simulink model "full_maneuver_platoon_new_strategy"  (R2019a)
settings: Solver=VariableStepAuto  StartTime=0.0  StopTime=70  FixedStep=0.1  MaxStep=0.05  RelTol=1e-3
libraries: simulink x97, dspsigops x7, powerlib_meascontrol x7, autolibshared x7
(part 2 of 7)

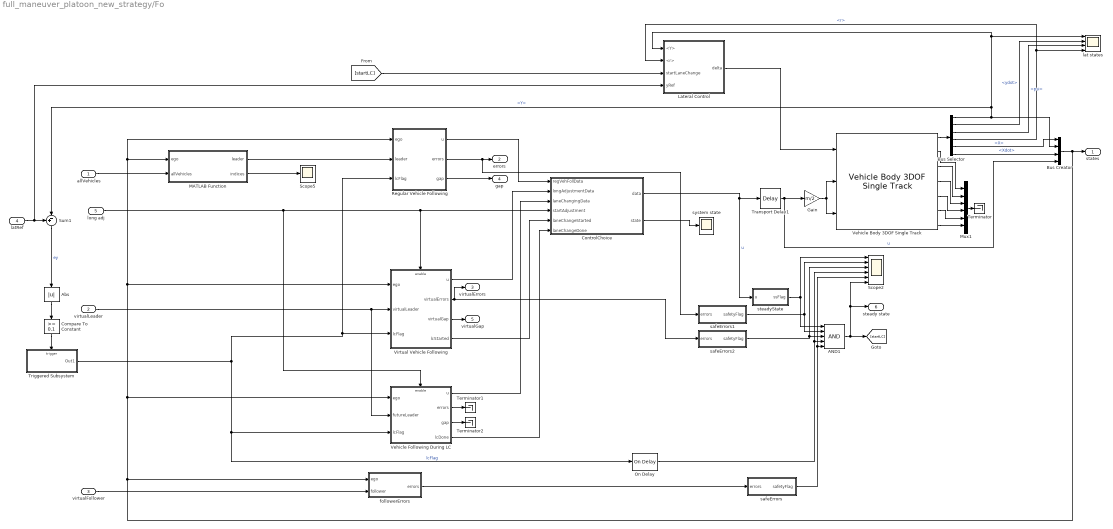
== system full_maneuver_platoon_new_strategy/Fo ==
  allVehicles : Inport
  virtualLeader : Inport  Port=2
  virtualFollower : Inport  Port=3
  latRef : Inport  Port=4
  long adj : Inport  Port=5
  AND1 : Logic  Inputs=5  IconShape=distinctive  AllPortsSameDT=off  OutDataTypeStr=boolean
  Abs : Abs
  Bus Creator : BusCreator  Inputs=4  OutDataTypeStr=Bus: vehStatesBus  NonVirtualBus=on
  Bus Selector : BusSelector  OutputSignals=InertFrm.Cg.Disp.Y,BdyFrm.Cg.Vel.ydot,InertFrm.Cg.Ang.psi,BdyFrm.Cg.AngVel.r,InertFrm.RearAxl.Disp.X,InertFrm.RearAxl.Vel.Xdot
  Compare To Constant : simulink/Logic and Bit Operations/Compare To Constant  relop=>=  const=0.1  OutDataTypeStr=boolean
  ControlChoice : Stateflow chart  BlockKeywords=__PRM__SERIALIZED__DATA__:Stateflow Chart,Stateflow Diagram  TreatAsAtomicUnit=on
  Gain : Gain  Gain=m/2
  Lateral Control : Subsystem
  MATLAB Function : MATLAB Function  TreatAsAtomicUnit=on
  Mux1 : Mux  Inputs=6
  On Delay : powerlib_meascontrol/Logic/On Delay  DelayType=On delay  delay=1  ic=0  Ts=0
      settings: SourceProductName=Simscape Electrical
  Regular Vehicle Following : Subsystem
  Scope2 : Scope  NumInputPorts=6
  Scope5 : Scope
  Sum1 : Sum  Inputs=+-|
  Terminator : Terminator
  Terminator1 : Terminator
  Terminator2 : Terminator
  Transport Delay1 : TransportDelay  DelayTime=0.01
  Triggered Subsystem : Subsystem  TreatAsAtomicUnit=on
  Vehicle Body 3DOF Single Track : autolibshared/Vehicle Body 3DOF Single Track  trackMode=Single (bicycle)  inputMode=External longitudinal forces  frontSteerMode=on  rearSteerMode=off  windMode=off  muMode=off  extFMode=off  extMMode=off  extXo=off  extpsio=off  extxdoto=off  extro=off  extYo=off  extTamb=off  extydoto=off  aMode=2  NF=2  NR=2  m=m  a=lf  b=lr  h=0.35  X_o=x0  xdot_o=vx0  CalphaMode=off  sigmaMode=on  d=0  w=[1.4,1.4]  Cy_f=12e3  Cy_r=11e3  sigma_f=.1  sigma_r=.1  alpha_f_brk=[-.1 .1]  Cy_f_data=[-9e3 9e3]  alpha_r_brk=[-.1 .1]  Cy_r_data=[-9e3 9e3]  Y_o=y0  ydot_o=0  Izz=4000  psi_o=0  r_o=0  Af=2  Cd=.3  Cl=.1  Cpm=.1  beta_w=[0:0.01:0.3]  Cs=[0:0.03:0.9]  Cym=[0:0.01:0.3]  Pabs=101325  Tair=273  g=9.81  mu=1  xdot_tol=.01  Fznom=5000  Fxtire_sat=7e4  Fytire_sat=7e4  longOff=0  latOff=0  vertOff=0  wrapAng=off
      settings: SourceProductName=Powertrain Blockset  SourceProductBaseCode=PW
  Vehicle Following During LC : Subsystem  TreatAsAtomicUnit=on
  Virtual Vehicle Following : Subsystem  TreatAsAtomicUnit=on
  followerErrors : Subsystem
  lat states : Scope  NumInputPorts=4
  safeErrors : Subsystem
  safeErrors1 : Subsystem
  safeErrors2 : Subsystem
  steadyState : Subsystem
  system state : Scope
  states : Outport
  errors : Outport  Port=2
  virtualErrors : Outport  Port=3
  gap : Outport  Port=4
  virtualGap : Outport  Port=5
  steady state : Outport  Port=6
  wires:
  Virtual Vehicle Following/2(virtualErrors) -> safeErrors2/1(errors), virtualErrors/1
  Sum1/1 -> Abs/1  "ey"
  Transport Delay1/1 -> Gain/1, Bus Creator/4  "u"
  virtualLeader/1 -> Vehicle Following During LC/2(futureLeader), Virtual Vehicle Following/2(virtualLeader)
  On Delay/1 -> Scope2/4, AND1/4
  long adj/1 -> Vehicle Following During LC/Enable, Virtual Vehicle Following/Enable, ControlChoice/4(startAdjustment)
  AND1/1 -> Scope2/6, steady state/1, [startLC]
  Bus Creator/1 -> states/1, Regular Vehicle Following/1(ego), MATLAB Function/1(ego), Virtual Vehicle Following/1(ego), Vehicle Following During LC/1(ego), followerErrors/1(ego)
  ControlChoice/1(data) -> Transport Delay1/1, steadyState/1(u)  "u"
  latRef/1 -> Lateral Control/4(yRef), Sum1/1
  Bus Selector/4 -> Lateral Control/2(<r>), lat states/4  "<r>"
  Bus Selector/3 -> lat states/3  "<psi>"
  Bus Selector/2 -> lat states/2  "<ydot>"
  Bus Selector/1 -> Lateral Control/1(<Y>), lat states/1, Sum1/2, Bus Creator/2  "<Y>"
  Mux1/1 -> Terminator/1
  Vehicle Body 3DOF Single Track/7 -> Mux1/6
  Vehicle Body 3DOF Single Track/6 -> Mux1/5
  Vehicle Body 3DOF Single Track/5 -> Mux1/4
  Vehicle Body 3DOF Single Track/2 -> Mux1/1
  Vehicle Body 3DOF Single Track/3 -> Mux1/2
  Vehicle Body 3DOF Single Track/4 -> Mux1/3
  Vehicle Body 3DOF Single Track/1 -> Bus Selector/1
  Gain/1 -> Vehicle Body 3DOF Single Track/2, Vehicle Body 3DOF Single Track/3
  Bus Selector/5 -> Bus Creator/1  "<X>"
  Bus Selector/6 -> Bus Creator/3  "<Xdot>"
  Triggered Subsystem/1(Out1) -> On Delay/1, Vehicle Following During LC/3(lcFlag), Regular Vehicle Following/3(lcFlag), Virtual Vehicle Following/3(lcFlag)  "lcFlag"
  Abs/1 -> Compare To Constant/1
  Compare To Constant/1 -> Triggered Subsystem/Trigger
  allVehicles/1 -> MATLAB Function/2(allVehicles)
  MATLAB Function/1(leader) -> Regular Vehicle Following/2(leader)
  safeErrors/1(safetyFlag) -> Scope2/5, AND1/5
  followerErrors/1(errors) -> safeErrors/1(errors)
  safeErrors1/1(safetyFlag) -> AND1/2, Scope2/2
  safeErrors2/1(safetyFlag) -> AND1/3, Scope2/3
  steadyState/1(ssFlag) -> AND1/1, Scope2/1
  virtualFollower/1 -> followerErrors/2(follower)
  MATLAB Function/2(indices) -> Scope5/1
  Regular Vehicle Following/3(gap) -> gap/1
  Regular Vehicle Following/1(u) -> ControlChoice/1(regVehFollData)
  Virtual Vehicle Following/1(u) -> ControlChoice/2(longAdjustmentData)
  Regular Vehicle Following/2(errors) -> safeErrors1/1(errors), errors/1
  [startLC] -> Lateral Control/3(startLaneChange)
  Lateral Control/1(delta) -> Vehicle Body 3DOF Single Track/1
  Virtual Vehicle Following/4(lcStarted) -> ControlChoice/5(laneChangeStarted)
  ControlChoice/2(state) -> system state/1
  Vehicle Following During LC/1(u) -> ControlChoice/3(laneChangingData)
  Vehicle Following During LC/4(lcDone) -> ControlChoice/6(laneChangeDone)
  Vehicle Following During LC/2(errors) -> Terminator1/1
  Vehicle Following During LC/3(gap) -> Terminator2/1
  Virtual Vehicle Following/3(virtualGap) -> virtualGap/1

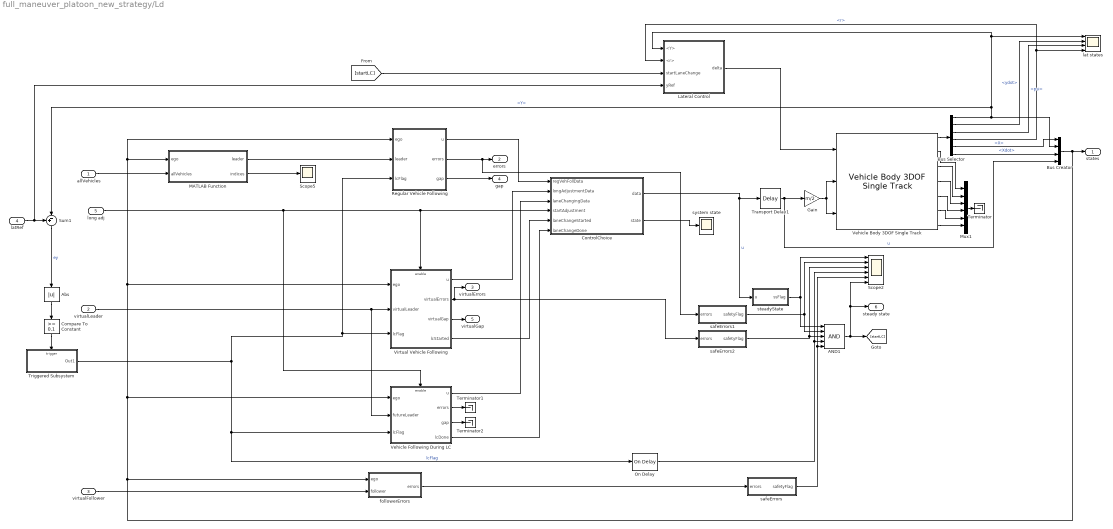
== system full_maneuver_platoon_new_strategy/Ld ==
  allVehicles : Inport
  virtualLeader : Inport  Port=2
  virtualFollower : Inport  Port=3
  latRef : Inport  Port=4
  long adj : Inport  Port=5
  AND1 : Logic  Inputs=5  IconShape=distinctive  AllPortsSameDT=off  OutDataTypeStr=boolean
  Abs : Abs
  Bus Creator : BusCreator  Inputs=4  OutDataTypeStr=Bus: vehStatesBus  NonVirtualBus=on
  Bus Selector : BusSelector  OutputSignals=InertFrm.Cg.Disp.Y,BdyFrm.Cg.Vel.ydot,InertFrm.Cg.Ang.psi,BdyFrm.Cg.AngVel.r,InertFrm.RearAxl.Disp.X,InertFrm.RearAxl.Vel.Xdot
  Compare To Constant : simulink/Logic and Bit Operations/Compare To Constant  relop=>=  const=0.1  OutDataTypeStr=boolean
  ControlChoice : Stateflow chart  BlockKeywords=__PRM__SERIALIZED__DATA__:Stateflow Chart,Stateflow Diagram  TreatAsAtomicUnit=on
  Gain : Gain  Gain=m/2
  Lateral Control : Subsystem
  MATLAB Function : MATLAB Function  TreatAsAtomicUnit=on
  Mux1 : Mux  Inputs=6
  On Delay : powerlib_meascontrol/Logic/On Delay  DelayType=On delay  delay=1  ic=0  Ts=0
      settings: SourceProductName=Simscape Electrical
  Regular Vehicle Following : Subsystem
  Scope2 : Scope  NumInputPorts=6
  Scope5 : Scope
  Sum1 : Sum  Inputs=+-|
  Terminator : Terminator
  Terminator1 : Terminator
  Terminator2 : Terminator
  Transport Delay1 : TransportDelay  DelayTime=0.01
  Triggered Subsystem : Subsystem  TreatAsAtomicUnit=on
  Vehicle Body 3DOF Single Track : autolibshared/Vehicle Body 3DOF Single Track  trackMode=Single (bicycle)  inputMode=External longitudinal forces  frontSteerMode=on  rearSteerMode=off  windMode=off  muMode=off  extFMode=off  extMMode=off  extXo=off  extpsio=off  extxdoto=off  extro=off  extYo=off  extTamb=off  extydoto=off  aMode=2  NF=2  NR=2  m=m  a=lf  b=lr  h=0.35  X_o=x0  xdot_o=vx0  CalphaMode=off  sigmaMode=on  d=0  w=[1.4,1.4]  Cy_f=12e3  Cy_r=11e3  sigma_f=.1  sigma_r=.1  alpha_f_brk=[-.1 .1]  Cy_f_data=[-9e3 9e3]  alpha_r_brk=[-.1 .1]  Cy_r_data=[-9e3 9e3]  Y_o=y0  ydot_o=0  Izz=4000  psi_o=0  r_o=0  Af=2  Cd=.3  Cl=.1  Cpm=.1  beta_w=[0:0.01:0.3]  Cs=[0:0.03:0.9]  Cym=[0:0.01:0.3]  Pabs=101325  Tair=273  g=9.81  mu=1  xdot_tol=.01  Fznom=5000  Fxtire_sat=7e4  Fytire_sat=7e4  longOff=0  latOff=0  vertOff=0  wrapAng=off
      settings: SourceProductName=Powertrain Blockset  SourceProductBaseCode=PW
  Vehicle Following During LC : Subsystem  TreatAsAtomicUnit=on
  Virtual Vehicle Following : Subsystem  TreatAsAtomicUnit=on
  followerErrors : Subsystem
  lat states : Scope  NumInputPorts=4
  safeErrors : Subsystem
  safeErrors1 : Subsystem
  safeErrors2 : Subsystem
  steadyState : Subsystem
  system state : Scope
  states : Outport
  errors : Outport  Port=2
  virtualErrors : Outport  Port=3
  gap : Outport  Port=4
  virtualGap : Outport  Port=5
  steady state : Outport  Port=6
  wires:
  Virtual Vehicle Following/2(virtualErrors) -> safeErrors2/1(errors), virtualErrors/1
  Sum1/1 -> Abs/1  "ey"
  Transport Delay1/1 -> Gain/1, Bus Creator/4  "u"
  virtualLeader/1 -> Vehicle Following During LC/2(futureLeader), Virtual Vehicle Following/2(virtualLeader)
  On Delay/1 -> Scope2/4, AND1/4
  long adj/1 -> Vehicle Following During LC/Enable, Virtual Vehicle Following/Enable, ControlChoice/4(startAdjustment)
  AND1/1 -> Scope2/6, steady state/1, [startLC]
  Bus Creator/1 -> states/1, Regular Vehicle Following/1(ego), MATLAB Function/1(ego), Virtual Vehicle Following/1(ego), Vehicle Following During LC/1(ego), followerErrors/1(ego)
  ControlChoice/1(data) -> Transport Delay1/1, steadyState/1(u)  "u"
  latRef/1 -> Lateral Control/4(yRef), Sum1/1
  Bus Selector/4 -> Lateral Control/2(<r>), lat states/4  "<r>"
  Bus Selector/3 -> lat states/3  "<psi>"
  Bus Selector/2 -> lat states/2  "<ydot>"
  Bus Selector/1 -> Lateral Control/1(<Y>), lat states/1, Sum1/2, Bus Creator/2  "<Y>"
  Mux1/1 -> Terminator/1
  Vehicle Body 3DOF Single Track/7 -> Mux1/6
  Vehicle Body 3DOF Single Track/6 -> Mux1/5
  Vehicle Body 3DOF Single Track/5 -> Mux1/4
  Vehicle Body 3DOF Single Track/2 -> Mux1/1
  Vehicle Body 3DOF Single Track/3 -> Mux1/2
  Vehicle Body 3DOF Single Track/4 -> Mux1/3
  Vehicle Body 3DOF Single Track/1 -> Bus Selector/1
  Gain/1 -> Vehicle Body 3DOF Single Track/2, Vehicle Body 3DOF Single Track/3
  Bus Selector/5 -> Bus Creator/1  "<X>"
  Bus Selector/6 -> Bus Creator/3  "<Xdot>"
  Triggered Subsystem/1(Out1) -> On Delay/1, Vehicle Following During LC/3(lcFlag), Regular Vehicle Following/3(lcFlag), Virtual Vehicle Following/3(lcFlag)  "lcFlag"
  Abs/1 -> Compare To Constant/1
  Compare To Constant/1 -> Triggered Subsystem/Trigger
  allVehicles/1 -> MATLAB Function/2(allVehicles)
  MATLAB Function/1(leader) -> Regular Vehicle Following/2(leader)
  safeErrors/1(safetyFlag) -> Scope2/5, AND1/5
  followerErrors/1(errors) -> safeErrors/1(errors)
  safeErrors1/1(safetyFlag) -> AND1/2, Scope2/2
  safeErrors2/1(safetyFlag) -> AND1/3, Scope2/3
  steadyState/1(ssFlag) -> AND1/1, Scope2/1
  virtualFollower/1 -> followerErrors/2(follower)
  MATLAB Function/2(indices) -> Scope5/1
  Regular Vehicle Following/3(gap) -> gap/1
  Regular Vehicle Following/1(u) -> ControlChoice/1(regVehFollData)
  Virtual Vehicle Following/1(u) -> ControlChoice/2(longAdjustmentData)
  Regular Vehicle Following/2(errors) -> safeErrors1/1(errors), errors/1
  [startLC] -> Lateral Control/3(startLaneChange)
  Lateral Control/1(delta) -> Vehicle Body 3DOF Single Track/1
  Virtual Vehicle Following/4(lcStarted) -> ControlChoice/5(laneChangeStarted)
  ControlChoice/2(state) -> system state/1
  Vehicle Following During LC/1(u) -> ControlChoice/3(laneChangingData)
  Vehicle Following During LC/4(lcDone) -> ControlChoice/6(laneChangeDone)
  Vehicle Following During LC/2(errors) -> Terminator1/1
  Vehicle Following During LC/3(gap) -> Terminator2/1
  Virtual Vehicle Following/3(virtualGap) -> virtualGap/1

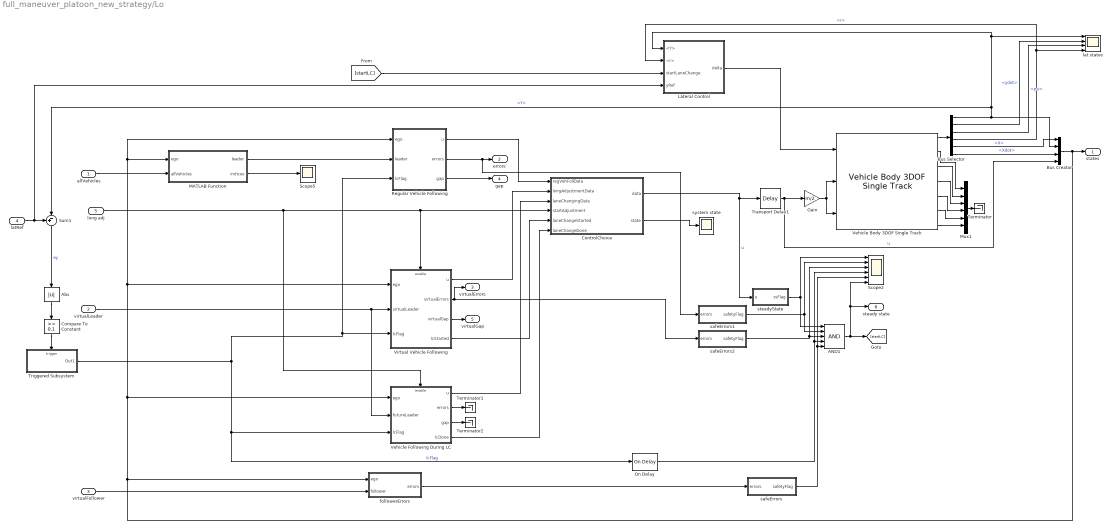
== system full_maneuver_platoon_new_strategy/Lo ==
  allVehicles : Inport
  virtualLeader : Inport  Port=2
  virtualFollower : Inport  Port=3
  latRef : Inport  Port=4
  long adj : Inport  Port=5
  AND1 : Logic  Inputs=5  IconShape=distinctive  AllPortsSameDT=off  OutDataTypeStr=boolean
  Abs : Abs
  Bus Creator : BusCreator  Inputs=4  OutDataTypeStr=Bus: vehStatesBus  NonVirtualBus=on
  Bus Selector : BusSelector  OutputSignals=InertFrm.Cg.Disp.Y,BdyFrm.Cg.Vel.ydot,InertFrm.Cg.Ang.psi,BdyFrm.Cg.AngVel.r,InertFrm.RearAxl.Disp.X,InertFrm.RearAxl.Vel.Xdot
  Compare To Constant : simulink/Logic and Bit Operations/Compare To Constant  relop=>=  const=0.1  OutDataTypeStr=boolean
  ControlChoice : Stateflow chart  BlockKeywords=__PRM__SERIALIZED__DATA__:Stateflow Chart,Stateflow Diagram  TreatAsAtomicUnit=on
  Gain : Gain  Gain=m/2
  Lateral Control : Subsystem
  MATLAB Function : MATLAB Function  TreatAsAtomicUnit=on
  Mux1 : Mux  Inputs=6
  On Delay : powerlib_meascontrol/Logic/On Delay  DelayType=On delay  delay=1  ic=0  Ts=0
      settings: SourceProductName=Simscape Electrical
  Regular Vehicle Following : Subsystem
  Scope2 : Scope  NumInputPorts=6
  Scope5 : Scope
  Sum1 : Sum  Inputs=+-|
  Terminator : Terminator
  Terminator1 : Terminator
  Terminator2 : Terminator
  Transport Delay1 : TransportDelay  DelayTime=0.01
  Triggered Subsystem : Subsystem  TreatAsAtomicUnit=on
  Vehicle Body 3DOF Single Track : autolibshared/Vehicle Body 3DOF Single Track  trackMode=Single (bicycle)  inputMode=External longitudinal forces  frontSteerMode=on  rearSteerMode=off  windMode=off  muMode=off  extFMode=off  extMMode=off  extXo=off  extpsio=off  extxdoto=off  extro=off  extYo=off  extTamb=off  extydoto=off  aMode=2  NF=2  NR=2  m=m  a=lf  b=lr  h=0.35  X_o=x0  xdot_o=vx0  CalphaMode=off  sigmaMode=on  d=0  w=[1.4,1.4]  Cy_f=12e3  Cy_r=11e3  sigma_f=.1  sigma_r=.1  alpha_f_brk=[-.1 .1]  Cy_f_data=[-9e3 9e3]  alpha_r_brk=[-.1 .1]  Cy_r_data=[-9e3 9e3]  Y_o=y0  ydot_o=0  Izz=4000  psi_o=0  r_o=0  Af=2  Cd=.3  Cl=.1  Cpm=.1  beta_w=[0:0.01:0.3]  Cs=[0:0.03:0.9]  Cym=[0:0.01:0.3]  Pabs=101325  Tair=273  g=9.81  mu=1  xdot_tol=.01  Fznom=5000  Fxtire_sat=7e4  Fytire_sat=7e4  longOff=0  latOff=0  vertOff=0  wrapAng=off
      settings: SourceProductName=Powertrain Blockset  SourceProductBaseCode=PW
  Vehicle Following During LC : Subsystem  TreatAsAtomicUnit=on
  Virtual Vehicle Following : Subsystem  TreatAsAtomicUnit=on
  followerErrors : Subsystem
  lat states : Scope  NumInputPorts=4
  safeErrors : Subsystem
  safeErrors1 : Subsystem
  safeErrors2 : Subsystem
  steadyState : Subsystem
  system state : Scope
  states : Outport
  errors : Outport  Port=2
  virtualErrors : Outport  Port=3
  gap : Outport  Port=4
  virtualGap : Outport  Port=5
  steady state : Outport  Port=6
  wires:
  Virtual Vehicle Following/3(virtualGap) -> virtualGap/1
  Vehicle Following During LC/3(gap) -> Terminator2/1
  Vehicle Following During LC/2(errors) -> Terminator1/1
  Vehicle Following During LC/4(lcDone) -> ControlChoice/6(laneChangeDone)
  Vehicle Following During LC/1(u) -> ControlChoice/3(laneChangingData)
  ControlChoice/2(state) -> system state/1
  Virtual Vehicle Following/4(lcStarted) -> ControlChoice/5(laneChangeStarted)
  Lateral Control/1(delta) -> Vehicle Body 3DOF Single Track/1
  [startLC] -> Lateral Control/3(startLaneChange)
  Regular Vehicle Following/2(errors) -> errors/1, safeErrors1/1(errors)
  Virtual Vehicle Following/1(u) -> ControlChoice/2(longAdjustmentData)
  Regular Vehicle Following/1(u) -> ControlChoice/1(regVehFollData)
  Regular Vehicle Following/3(gap) -> gap/1
  MATLAB Function/2(indices) -> Scope5/1
  virtualFollower/1 -> followerErrors/2(follower)
  steadyState/1(ssFlag) -> Scope2/1, AND1/1
  safeErrors2/1(safetyFlag) -> Scope2/3, AND1/3
  safeErrors1/1(safetyFlag) -> Scope2/2, AND1/2
  followerErrors/1(errors) -> safeErrors/1(errors)
  safeErrors/1(safetyFlag) -> AND1/5, Scope2/5
  MATLAB Function/1(leader) -> Regular Vehicle Following/2(leader)
  allVehicles/1 -> MATLAB Function/2(allVehicles)
  Compare To Constant/1 -> Triggered Subsystem/Trigger
  Abs/1 -> Compare To Constant/1
  Triggered Subsystem/1(Out1) -> Virtual Vehicle Following/3(lcFlag), Regular Vehicle Following/3(lcFlag), Vehicle Following During LC/3(lcFlag), On Delay/1  "lcFlag"
  Bus Selector/6 -> Bus Creator/3  "<Xdot>"
  Bus Selector/5 -> Bus Creator/1  "<X>"
  Gain/1 -> Vehicle Body 3DOF Single Track/3, Vehicle Body 3DOF Single Track/2
  Vehicle Body 3DOF Single Track/1 -> Bus Selector/1
  Vehicle Body 3DOF Single Track/4 -> Mux1/3
  Vehicle Body 3DOF Single Track/3 -> Mux1/2
  Vehicle Body 3DOF Single Track/2 -> Mux1/1
  Vehicle Body 3DOF Single Track/5 -> Mux1/4
  Vehicle Body 3DOF Single Track/6 -> Mux1/5
  Vehicle Body 3DOF Single Track/7 -> Mux1/6
  Mux1/1 -> Terminator/1
  Bus Selector/1 -> Bus Creator/2, Sum1/2, lat states/1, Lateral Control/1(<Y>)  "<Y>"
  Bus Selector/2 -> lat states/2  "<ydot>"
  Bus Selector/3 -> lat states/3  "<psi>"
  Bus Selector/4 -> lat states/4, Lateral Control/2(<r>)  "<r>"
  latRef/1 -> Sum1/1, Lateral Control/4(yRef)
  ControlChoice/1(data) -> steadyState/1(u), Transport Delay1/1  "u"
  Bus Creator/1 -> followerErrors/1(ego), Vehicle Following During LC/1(ego), Virtual Vehicle Following/1(ego), MATLAB Function/1(ego), Regular Vehicle Following/1(ego), states/1
  AND1/1 -> [startLC], steady state/1, Scope2/6
  long adj/1 -> ControlChoice/4(startAdjustment), Virtual Vehicle Following/Enable, Vehicle Following During LC/Enable
  On Delay/1 -> AND1/4, Scope2/4
  virtualLeader/1 -> Virtual Vehicle Following/2(virtualLeader), Vehicle Following During LC/2(futureLeader)
  Transport Delay1/1 -> Bus Creator/4, Gain/1  "u"
  Sum1/1 -> Abs/1  "ey"
  Virtual Vehicle Following/2(virtualErrors) -> virtualErrors/1, safeErrors2/1(errors)

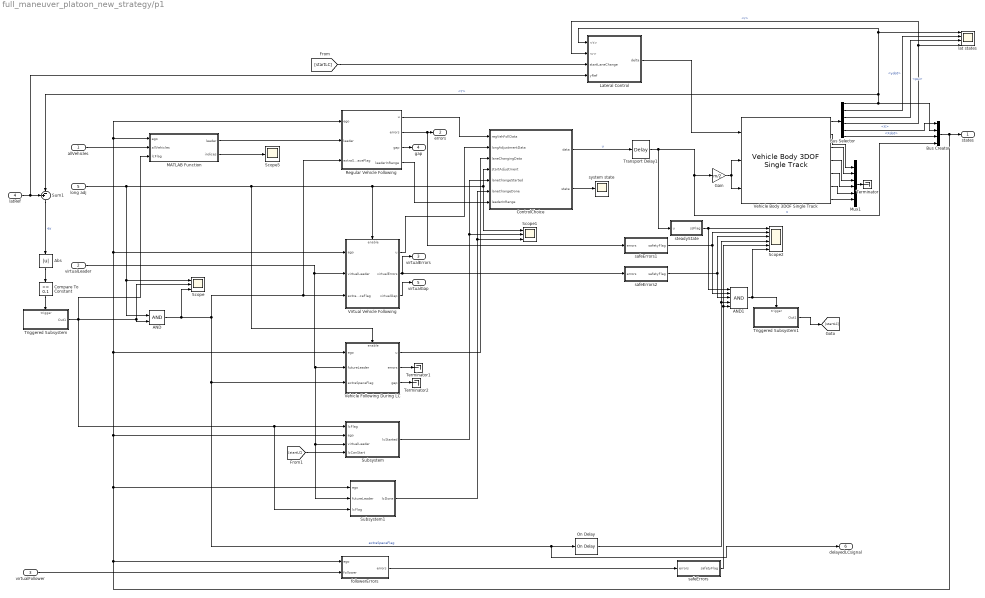
== system full_maneuver_platoon_new_strategy/p1 ==
  allVehicles : Inport
  virtualLeader : Inport  Port=2
  virtualFollower : Inport  Port=3
  latRef : Inport  Port=4
  long adj : Inport  Port=5
  AND : Logic  IconShape=distinctive  AllPortsSameDT=off  OutDataTypeStr=boolean
  AND1 : Logic  Inputs=5  IconShape=distinctive  AllPortsSameDT=off  OutDataTypeStr=boolean
  Abs : Abs
  Bus Creator : BusCreator  Inputs=4  OutDataTypeStr=Bus: vehStatesBus  NonVirtualBus=on
  Bus Selector : BusSelector  OutputSignals=InertFrm.Cg.Disp.Y,BdyFrm.Cg.Vel.ydot,InertFrm.Cg.Ang.psi,BdyFrm.Cg.AngVel.r,InertFrm.RearAxl.Disp.X,InertFrm.RearAxl.Vel.Xdot
  Compare To Constant : simulink/Logic and Bit Operations/Compare To Constant  relop=>=  const=0.1  OutDataTypeStr=boolean
  ControlChoice : Stateflow chart  BlockKeywords=__PRM__SERIALIZED__DATA__:Stateflow Chart,Stateflow Diagram  TreatAsAtomicUnit=on
  Gain : Gain  Gain=m/2
  Lateral Control : Subsystem
  MATLAB Function : MATLAB Function  TreatAsAtomicUnit=on
  Mux1 : Mux  Inputs=6
  On Delay : powerlib_meascontrol/Logic/On Delay  DelayType=On delay  delay=1  ic=0  Ts=0
      settings: SourceProductName=Simscape Electrical
  Regular Vehicle Following : Subsystem
  Scope : Scope  NumInputPorts=3
  Scope1 : Scope  NumInputPorts=3
  Scope2 : Scope  NumInputPorts=6
  Scope5 : Scope
  Subsystem : Subsystem
  Subsystem1 : Subsystem
  Sum1 : Sum  Inputs=+-|
  Terminator : Terminator
  Terminator1 : Terminator
  Terminator2 : Terminator
  Transport Delay1 : TransportDelay  DelayTime=0.01
  Triggered Subsystem : Subsystem  TreatAsAtomicUnit=on
  Triggered Subsystem1 : Subsystem  TreatAsAtomicUnit=on
  Vehicle Body 3DOF Single Track : autolibshared/Vehicle Body 3DOF Single Track  trackMode=Single (bicycle)  inputMode=External longitudinal forces  frontSteerMode=on  rearSteerMode=off  windMode=off  muMode=off  extFMode=off  extMMode=off  extXo=off  extpsio=off  extxdoto=off  extro=off  extYo=off  extTamb=off  extydoto=off  aMode=2  NF=2  NR=2  m=m  a=lf  b=lr  h=0.35  X_o=x0  xdot_o=vx0  CalphaMode=off  sigmaMode=on  d=0  w=[1.4,1.4]  Cy_f=12e3  Cy_r=11e3  sigma_f=.1  sigma_r=.1  alpha_f_brk=[-.1 .1]  Cy_f_data=[-9e3 9e3]  alpha_r_brk=[-.1 .1]  Cy_r_data=[-9e3 9e3]  Y_o=y0  ydot_o=0  Izz=4000  psi_o=0  r_o=0  Af=2  Cd=.3  Cl=.1  Cpm=.1  beta_w=[0:0.01:0.3]  Cs=[0:0.03:0.9]  Cym=[0:0.01:0.3]  Pabs=101325  Tair=273  g=9.81  mu=1  xdot_tol=.01  Fznom=5000  Fxtire_sat=7e4  Fytire_sat=7e4  longOff=0  latOff=0  vertOff=0  wrapAng=off
      settings: SourceProductName=Powertrain Blockset  SourceProductBaseCode=PW
  Vehicle Following During LC : Subsystem  TreatAsAtomicUnit=on
  Virtual Vehicle Following : Subsystem  TreatAsAtomicUnit=on
  followerErrors : Subsystem
  lat states : Scope  NumInputPorts=4
  safeErrors : Subsystem
  safeErrors1 : Subsystem
  safeErrors2 : Subsystem
  steadyState : Subsystem
  system state : Scope
  states : Outport
  errors : Outport  Port=2
  virtualErrors : Outport  Port=3
  gap : Outport  Port=4
  virtualGap : Outport  Port=5
  delayedLCsignal : Outport  Port=6
  wires:
  Regular Vehicle Following/4(leaderInRange) -> ControlChoice/7(leaderInRange)
  Triggered Subsystem1/1(Out1) -> [startLC]
  Triggered Subsystem/1(Out1) -> Scope/2, AND/2, Subsystem/1(lcFlag), Subsystem1/3(lcFlag), MATLAB Function/3(lcFlag)
  [startLC] -> Subsystem/4(lcCanStart)
  Virtual Vehicle Following/3(virtualGap) -> virtualGap/1
  Vehicle Following During LC/3(gap) -> Terminator2/1
  Vehicle Following During LC/2(errors) -> Terminator1/1
  Subsystem1/1(lcDone) -> ControlChoice/6(laneChangeDone), Scope1/3
  Vehicle Following During LC/1(u) -> ControlChoice/3(laneChangingData)
  ControlChoice/2(state) -> system state/1
  Subsystem/1(lcStarted) -> ControlChoice/5(laneChangeStarted), Scope1/2
  Lateral Control/1(delta) -> Vehicle Body 3DOF Single Track/1
  [startLC] -> Lateral Control/3(startLaneChange)
  Regular Vehicle Following/2(errors) -> errors/1, safeErrors1/1(errors)
  Virtual Vehicle Following/1(u) -> ControlChoice/2(longAdjustmentData)
  Regular Vehicle Following/1(u) -> ControlChoice/1(regVehFollData)
  Regular Vehicle Following/3(gap) -> gap/1
  MATLAB Function/2(indices) -> Scope5/1
  virtualFollower/1 -> followerErrors/2(follower)
  steadyState/1(ssFlag) -> Scope2/1, AND1/1
  safeErrors2/1(safetyFlag) -> AND1/3, Scope2/3
  safeErrors1/1(safetyFlag) -> Scope2/2, AND1/2
  followerErrors/1(errors) -> safeErrors/1(errors)
  safeErrors/1(safetyFlag) -> AND1/5, Scope2/5
  MATLAB Function/1(leader) -> Regular Vehicle Following/2(leader)
  allVehicles/1 -> MATLAB Function/2(allVehicles)
  Compare To Constant/1 -> Triggered Subsystem/Trigger
  Abs/1 -> Compare To Constant/1
  AND/1 -> Vehicle Following During LC/3(extraSpaceFlag), delayedLCsignal/1, On Delay/1, Virtual Vehicle Following/3(extraSpaceFlag), Regular Vehicle Following/3(extraSpaceFlag), Scope/3  "extraSpaceFlag"
  Bus Selector/6 -> Bus Creator/3  "<Xdot>"
  Bus Selector/5 -> Bus Creator/1  "<X>"
  Gain/1 -> Vehicle Body 3DOF Single Track/3, Vehicle Body 3DOF Single Track/2
  Vehicle Body 3DOF Single Track/1 -> Bus Selector/1
  Vehicle Body 3DOF Single Track/4 -> Mux1/3
  Vehicle Body 3DOF Single Track/3 -> Mux1/2
  Vehicle Body 3DOF Single Track/2 -> Mux1/1
  Vehicle Body 3DOF Single Track/5 -> Mux1/4
  Vehicle Body 3DOF Single Track/6 -> Mux1/5
  Vehicle Body 3DOF Single Track/7 -> Mux1/6
  Mux1/1 -> Terminator/1
  Bus Selector/1 -> Bus Creator/2, Sum1/2, lat states/1, Lateral Control/1(<Y>)  "<Y>"
  Bus Selector/2 -> lat states/2  "<ydot>"
  Bus Selector/3 -> lat states/3  "<psi>"
  Bus Selector/4 -> lat states/4, Lateral Control/2(<r>)  "<r>"
  latRef/1 -> Sum1/1, Lateral Control/4(yRef)
  ControlChoice/1(data) -> Transport Delay1/1  "u"
  Bus Creator/1 -> followerErrors/1(ego), Subsystem/2(ego), Vehicle Following During LC/1(ego), Virtual Vehicle Following/1(ego), MATLAB Function/1(ego), Regular Vehicle Following/1(ego), Subsystem1/1(ego), states/1
  AND1/1 -> Scope2/6, Triggered Subsystem1/Trigger
  long adj/1 -> AND/1, Scope/1, ControlChoice/4(startAdjustment), Scope1/1, Virtual Vehicle Following/Enable, Vehicle Following During LC/Enable
  On Delay/1 -> AND1/4, Scope2/4
  virtualLeader/1 -> Virtual Vehicle Following/2(virtualLeader), Vehicle Following During LC/2(futureLeader), Subsystem/3(virtualLeader), Subsystem1/2(futureLeader)
  Transport Delay1/1 -> Gain/1, Bus Creator/4, steadyState/1(u)  "u"
  Sum1/1 -> Abs/1  "ey"
  Virtual Vehicle Following/2(virtualErrors) -> safeErrors2/1(errors), virtualErrors/1

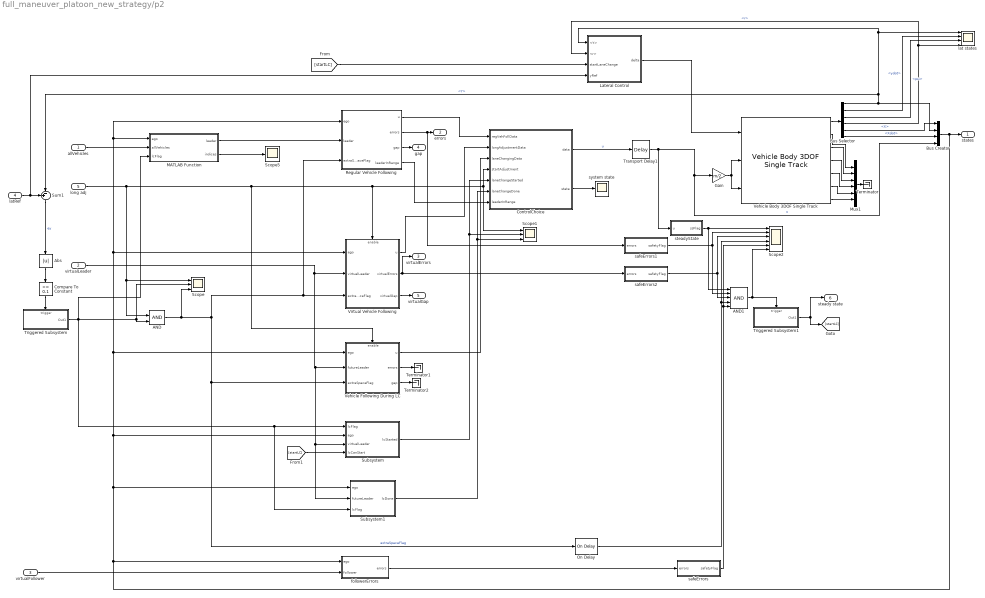
== system full_maneuver_platoon_new_strategy/p2 ==
  allVehicles : Inport
  virtualLeader : Inport  Port=2
  virtualFollower : Inport  Port=3
  latRef : Inport  Port=4
  long adj : Inport  Port=5
  AND : Logic  IconShape=distinctive  AllPortsSameDT=off  OutDataTypeStr=boolean
  AND1 : Logic  Inputs=5  IconShape=distinctive  AllPortsSameDT=off  OutDataTypeStr=boolean
  Abs : Abs
  Bus Creator : BusCreator  Inputs=4  OutDataTypeStr=Bus: vehStatesBus  NonVirtualBus=on
  Bus Selector : BusSelector  OutputSignals=InertFrm.Cg.Disp.Y,BdyFrm.Cg.Vel.ydot,InertFrm.Cg.Ang.psi,BdyFrm.Cg.AngVel.r,InertFrm.RearAxl.Disp.X,InertFrm.RearAxl.Vel.Xdot
  Compare To Constant : simulink/Logic and Bit Operations/Compare To Constant  relop=>=  const=0.1  OutDataTypeStr=boolean
  ControlChoice : Stateflow chart  BlockKeywords=__PRM__SERIALIZED__DATA__:Stateflow Chart,Stateflow Diagram  TreatAsAtomicUnit=on
  Gain : Gain  Gain=m/2
  Lateral Control : Subsystem
  MATLAB Function : MATLAB Function  TreatAsAtomicUnit=on
  Mux1 : Mux  Inputs=6
  On Delay : powerlib_meascontrol/Logic/On Delay  DelayType=On delay  delay=1  ic=0  Ts=0
      settings: SourceProductName=Simscape Electrical
  Regular Vehicle Following : Subsystem
  Scope : Scope  NumInputPorts=3
  Scope1 : Scope  NumInputPorts=3
  Scope2 : Scope  NumInputPorts=6
  Scope5 : Scope
  Subsystem : Subsystem
  Subsystem1 : Subsystem
  Sum1 : Sum  Inputs=+-|
  Terminator : Terminator
  Terminator1 : Terminator
  Terminator2 : Terminator
  Transport Delay1 : TransportDelay  DelayTime=0.01
  Triggered Subsystem : Subsystem  TreatAsAtomicUnit=on
  Triggered Subsystem1 : Subsystem  TreatAsAtomicUnit=on
  Vehicle Body 3DOF Single Track : autolibshared/Vehicle Body 3DOF Single Track  trackMode=Single (bicycle)  inputMode=External longitudinal forces  frontSteerMode=on  rearSteerMode=off  windMode=off  muMode=off  extFMode=off  extMMode=off  extXo=off  extpsio=off  extxdoto=off  extro=off  extYo=off  extTamb=off  extydoto=off  aMode=2  NF=2  NR=2  m=m  a=lf  b=lr  h=0.35  X_o=x0  xdot_o=vx0  CalphaMode=off  sigmaMode=on  d=0  w=[1.4,1.4]  Cy_f=12e3  Cy_r=11e3  sigma_f=.1  sigma_r=.1  alpha_f_brk=[-.1 .1]  Cy_f_data=[-9e3 9e3]  alpha_r_brk=[-.1 .1]  Cy_r_data=[-9e3 9e3]  Y_o=y0  ydot_o=0  Izz=4000  psi_o=0  r_o=0  Af=2  Cd=.3  Cl=.1  Cpm=.1  beta_w=[0:0.01:0.3]  Cs=[0:0.03:0.9]  Cym=[0:0.01:0.3]  Pabs=101325  Tair=273  g=9.81  mu=1  xdot_tol=.01  Fznom=5000  Fxtire_sat=7e4  Fytire_sat=7e4  longOff=0  latOff=0  vertOff=0  wrapAng=off
      settings: SourceProductName=Powertrain Blockset  SourceProductBaseCode=PW
  Vehicle Following During LC : Subsystem  TreatAsAtomicUnit=on
  Virtual Vehicle Following : Subsystem  TreatAsAtomicUnit=on
  followerErrors : Subsystem
  lat states : Scope  NumInputPorts=4
  safeErrors : Subsystem
  safeErrors1 : Subsystem
  safeErrors2 : Subsystem
  steadyState : Subsystem
  system state : Scope
  states : Outport
  errors : Outport  Port=2
  virtualErrors : Outport  Port=3
  gap : Outport  Port=4
  virtualGap : Outport  Port=5
  steady state : Outport  Port=6
  wires:
  Virtual Vehicle Following/2(virtualErrors) -> virtualErrors/1, safeErrors2/1(errors)
  Sum1/1 -> Abs/1  "ey"
  Transport Delay1/1 -> steadyState/1(u), Bus Creator/4, Gain/1  "u"
  virtualLeader/1 -> Subsystem1/2(futureLeader), Subsystem/3(virtualLeader), Vehicle Following During LC/2(futureLeader), Virtual Vehicle Following/2(virtualLeader)
  On Delay/1 -> Scope2/4, AND1/4
  long adj/1 -> Vehicle Following During LC/Enable, Virtual Vehicle Following/Enable, Scope1/1, ControlChoice/4(startAdjustment), Scope/1, AND/1
  AND1/1 -> Triggered Subsystem1/Trigger, Scope2/6
  Bus Creator/1 -> states/1, Subsystem1/1(ego), Regular Vehicle Following/1(ego), MATLAB Function/1(ego), Virtual Vehicle Following/1(ego), Vehicle Following During LC/1(ego), Subsystem/2(ego), followerErrors/1(ego)
  ControlChoice/1(data) -> Transport Delay1/1  "u"
  latRef/1 -> Lateral Control/4(yRef), Sum1/1
  Bus Selector/4 -> Lateral Control/2(<r>), lat states/4  "<r>"
  Bus Selector/3 -> lat states/3  "<psi>"
  Bus Selector/2 -> lat states/2  "<ydot>"
  Bus Selector/1 -> Lateral Control/1(<Y>), lat states/1, Sum1/2, Bus Creator/2  "<Y>"
  Mux1/1 -> Terminator/1
  Vehicle Body 3DOF Single Track/7 -> Mux1/6
  Vehicle Body 3DOF Single Track/6 -> Mux1/5
  Vehicle Body 3DOF Single Track/5 -> Mux1/4
  Vehicle Body 3DOF Single Track/2 -> Mux1/1
  Vehicle Body 3DOF Single Track/3 -> Mux1/2
  Vehicle Body 3DOF Single Track/4 -> Mux1/3
  Vehicle Body 3DOF Single Track/1 -> Bus Selector/1
  Gain/1 -> Vehicle Body 3DOF Single Track/2, Vehicle Body 3DOF Single Track/3
  Bus Selector/5 -> Bus Creator/1  "<X>"
  Bus Selector/6 -> Bus Creator/3  "<Xdot>"
  AND/1 -> Scope/3, Regular Vehicle Following/3(extraSpaceFlag), Virtual Vehicle Following/3(extraSpaceFlag), On Delay/1, Vehicle Following During LC/3(extraSpaceFlag)  "extraSpaceFlag"
  Abs/1 -> Compare To Constant/1
  Compare To Constant/1 -> Triggered Subsystem/Trigger
  allVehicles/1 -> MATLAB Function/2(allVehicles)
  MATLAB Function/1(leader) -> Regular Vehicle Following/2(leader)
  safeErrors/1(safetyFlag) -> Scope2/5, AND1/5
  followerErrors/1(errors) -> safeErrors/1(errors)
  safeErrors1/1(safetyFlag) -> AND1/2, Scope2/2
  safeErrors2/1(safetyFlag) -> Scope2/3, AND1/3
  steadyState/1(ssFlag) -> AND1/1, Scope2/1
  virtualFollower/1 -> followerErrors/2(follower)
  MATLAB Function/2(indices) -> Scope5/1
  Regular Vehicle Following/3(gap) -> gap/1
  Regular Vehicle Following/1(u) -> ControlChoice/1(regVehFollData)
  Virtual Vehicle Following/1(u) -> ControlChoice/2(longAdjustmentData)
  Regular Vehicle Following/2(errors) -> safeErrors1/1(errors), errors/1
  [startLC] -> Lateral Control/3(startLaneChange)
  Lateral Control/1(delta) -> Vehicle Body 3DOF Single Track/1
  Subsystem/1(lcStarted) -> Scope1/2, ControlChoice/5(laneChangeStarted)
  ControlChoice/2(state) -> system state/1
  Vehicle Following During LC/1(u) -> ControlChoice/3(laneChangingData)
  Subsystem1/1(lcDone) -> Scope1/3, ControlChoice/6(laneChangeDone)
  Vehicle Following During LC/2(errors) -> Terminator1/1
  Vehicle Following During LC/3(gap) -> Terminator2/1
  Virtual Vehicle Following/3(virtualGap) -> virtualGap/1
  [startLC] -> Subsystem/4(lcCanStart)
  Triggered Subsystem/1(Out1) -> MATLAB Function/3(lcFlag), Subsystem1/3(lcFlag), Subsystem/1(lcFlag), AND/2, Scope/2
  Triggered Subsystem1/1(Out1) -> steady state/1, [startLC]
  Regular Vehicle Following/4(leaderInRange) -> ControlChoice/7(leaderInRange)

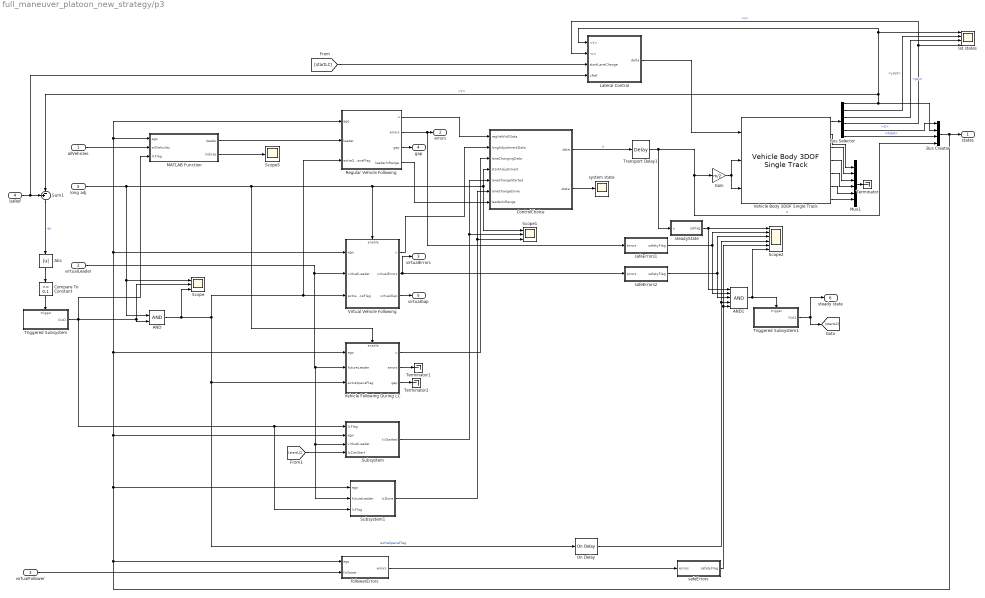
== system full_maneuver_platoon_new_strategy/p3 ==
  allVehicles : Inport
  virtualLeader : Inport  Port=2
  virtualFollower : Inport  Port=3
  latRef : Inport  Port=4
  long adj : Inport  Port=5
  AND : Logic  IconShape=distinctive  AllPortsSameDT=off  OutDataTypeStr=boolean
  AND1 : Logic  Inputs=5  IconShape=distinctive  AllPortsSameDT=off  OutDataTypeStr=boolean
  Abs : Abs
  Bus Creator : BusCreator  Inputs=4  OutDataTypeStr=Bus: vehStatesBus  NonVirtualBus=on
  Bus Selector : BusSelector  OutputSignals=InertFrm.Cg.Disp.Y,BdyFrm.Cg.Vel.ydot,InertFrm.Cg.Ang.psi,BdyFrm.Cg.AngVel.r,InertFrm.RearAxl.Disp.X,InertFrm.RearAxl.Vel.Xdot
  Compare To Constant : simulink/Logic and Bit Operations/Compare To Constant  relop=>=  const=0.1  OutDataTypeStr=boolean
  ControlChoice : Stateflow chart  BlockKeywords=__PRM__SERIALIZED__DATA__:Stateflow Chart,Stateflow Diagram  TreatAsAtomicUnit=on
  Gain : Gain  Gain=m/2
  Lateral Control : Subsystem
  MATLAB Function : MATLAB Function  TreatAsAtomicUnit=on
  Mux1 : Mux  Inputs=6
  On Delay : powerlib_meascontrol/Logic/On Delay  DelayType=On delay  delay=1  ic=0  Ts=0
      settings: SourceProductName=Simscape Electrical
  Regular Vehicle Following : Subsystem
  Scope : Scope  NumInputPorts=3
  Scope1 : Scope  NumInputPorts=3
  Scope2 : Scope  NumInputPorts=6
  Scope5 : Scope
  Subsystem : Subsystem
  Subsystem1 : Subsystem
  Sum1 : Sum  Inputs=+-|
  Terminator : Terminator
  Terminator1 : Terminator
  Terminator2 : Terminator
  Transport Delay1 : TransportDelay  DelayTime=0.01
  Triggered Subsystem : Subsystem  TreatAsAtomicUnit=on
  Triggered Subsystem1 : Subsystem  TreatAsAtomicUnit=on
  Vehicle Body 3DOF Single Track : autolibshared/Vehicle Body 3DOF Single Track  trackMode=Single (bicycle)  inputMode=External longitudinal forces  frontSteerMode=on  rearSteerMode=off  windMode=off  muMode=off  extFMode=off  extMMode=off  extXo=off  extpsio=off  extxdoto=off  extro=off  extYo=off  extTamb=off  extydoto=off  aMode=2  NF=2  NR=2  m=m  a=lf  b=lr  h=0.35  X_o=x0  xdot_o=vx0  CalphaMode=off  sigmaMode=on  d=0  w=[1.4,1.4]  Cy_f=12e3  Cy_r=11e3  sigma_f=.1  sigma_r=.1  alpha_f_brk=[-.1 .1]  Cy_f_data=[-9e3 9e3]  alpha_r_brk=[-.1 .1]  Cy_r_data=[-9e3 9e3]  Y_o=y0  ydot_o=0  Izz=4000  psi_o=0  r_o=0  Af=2  Cd=.3  Cl=.1  Cpm=.1  beta_w=[0:0.01:0.3]  Cs=[0:0.03:0.9]  Cym=[0:0.01:0.3]  Pabs=101325  Tair=273  g=9.81  mu=1  xdot_tol=.01  Fznom=5000  Fxtire_sat=7e4  Fytire_sat=7e4  longOff=0  latOff=0  vertOff=0  wrapAng=off
      settings: SourceProductName=Powertrain Blockset  SourceProductBaseCode=PW
  Vehicle Following During LC : Subsystem  TreatAsAtomicUnit=on
  Virtual Vehicle Following : Subsystem  TreatAsAtomicUnit=on
  followerErrors : Subsystem
  lat states : Scope  NumInputPorts=4
  safeErrors : Subsystem
  safeErrors1 : Subsystem
  safeErrors2 : Subsystem
  steadyState : Subsystem
  system state : Scope
  states : Outport
  errors : Outport  Port=2
  virtualErrors : Outport  Port=3
  gap : Outport  Port=4
  virtualGap : Outport  Port=5
  steady state : Outport  Port=6
  wires:
  Regular Vehicle Following/4(leaderInRange) -> ControlChoice/7(leaderInRange)
  Triggered Subsystem1/1(Out1) -> [startLC], steady state/1
  Triggered Subsystem/1(Out1) -> Scope/2, AND/2, Subsystem/1(lcFlag), Subsystem1/3(lcFlag), MATLAB Function/3(lcFlag)
  [startLC] -> Subsystem/4(lcCanStart)
  Virtual Vehicle Following/3(virtualGap) -> virtualGap/1
  Vehicle Following During LC/3(gap) -> Terminator2/1
  Vehicle Following During LC/2(errors) -> Terminator1/1
  Subsystem1/1(lcDone) -> ControlChoice/6(laneChangeDone), Scope1/3
  Vehicle Following During LC/1(u) -> ControlChoice/3(laneChangingData)
  ControlChoice/2(state) -> system state/1
  Subsystem/1(lcStarted) -> ControlChoice/5(laneChangeStarted), Scope1/2
  Lateral Control/1(delta) -> Vehicle Body 3DOF Single Track/1
  [startLC] -> Lateral Control/3(startLaneChange)
  Regular Vehicle Following/2(errors) -> errors/1, safeErrors1/1(errors)
  Virtual Vehicle Following/1(u) -> ControlChoice/2(longAdjustmentData)
  Regular Vehicle Following/1(u) -> ControlChoice/1(regVehFollData)
  Regular Vehicle Following/3(gap) -> gap/1
  MATLAB Function/2(indices) -> Scope5/1
  virtualFollower/1 -> followerErrors/2(follower)
  steadyState/1(ssFlag) -> Scope2/1, AND1/1
  safeErrors2/1(safetyFlag) -> AND1/3, Scope2/3
  safeErrors1/1(safetyFlag) -> Scope2/2, AND1/2
  followerErrors/1(errors) -> safeErrors/1(errors)
  safeErrors/1(safetyFlag) -> AND1/5, Scope2/5
  MATLAB Function/1(leader) -> Regular Vehicle Following/2(leader)
  allVehicles/1 -> MATLAB Function/2(allVehicles)
  Compare To Constant/1 -> Triggered Subsystem/Trigger
  Abs/1 -> Compare To Constant/1
  AND/1 -> Vehicle Following During LC/3(extraSpaceFlag), On Delay/1, Virtual Vehicle Following/3(extraSpaceFlag), Regular Vehicle Following/3(extraSpaceFlag), Scope/3  "extraSpaceFlag"
  Bus Selector/6 -> Bus Creator/3  "<Xdot>"
  Bus Selector/5 -> Bus Creator/1  "<X>"
  Gain/1 -> Vehicle Body 3DOF Single Track/3, Vehicle Body 3DOF Single Track/2
  Vehicle Body 3DOF Single Track/1 -> Bus Selector/1
  Vehicle Body 3DOF Single Track/4 -> Mux1/3
  Vehicle Body 3DOF Single Track/3 -> Mux1/2
  Vehicle Body 3DOF Single Track/2 -> Mux1/1
  Vehicle Body 3DOF Single Track/5 -> Mux1/4
  Vehicle Body 3DOF Single Track/6 -> Mux1/5
  Vehicle Body 3DOF Single Track/7 -> Mux1/6
  Mux1/1 -> Terminator/1
  Bus Selector/1 -> Bus Creator/2, Sum1/2, lat states/1, Lateral Control/1(<Y>)  "<Y>"
  Bus Selector/2 -> lat states/2  "<ydot>"
  Bus Selector/3 -> lat states/3  "<psi>"
  Bus Selector/4 -> lat states/4, Lateral Control/2(<r>)  "<r>"
  latRef/1 -> Sum1/1, Lateral Control/4(yRef)
  ControlChoice/1(data) -> Transport Delay1/1  "u"
  Bus Creator/1 -> followerErrors/1(ego), Subsystem/2(ego), Vehicle Following During LC/1(ego), Virtual Vehicle Following/1(ego), MATLAB Function/1(ego), Regular Vehicle Following/1(ego), Subsystem1/1(ego), states/1
  AND1/1 -> Scope2/6, Triggered Subsystem1/Trigger
  long adj/1 -> AND/1, Scope/1, ControlChoice/4(startAdjustment), Scope1/1, Virtual Vehicle Following/Enable, Vehicle Following During LC/Enable
  On Delay/1 -> AND1/4, Scope2/4
  virtualLeader/1 -> Virtual Vehicle Following/2(virtualLeader), Vehicle Following During LC/2(futureLeader), Subsystem/3(virtualLeader), Subsystem1/2(futureLeader)
  Transport Delay1/1 -> Gain/1, Bus Creator/4, steadyState/1(u)  "u"
  Sum1/1 -> Abs/1  "ey"
  Virtual Vehicle Following/2(virtualErrors) -> safeErrors2/1(errors), virtualErrors/1

== system full_maneuver_platoon_new_strategy/Fd/Lateral Control ==
  <Y> : Inport
  <r> : Inport  Port=2
  startLaneChange : Inport  Port=3
  yRef : Inport  Port=4
  Demux2 : Demux
  Full State Observer : Subsystem
  Gain1 : Gain  Gain=Klat  Multiplication=Matrix(K*u)
  Integrator : Integrator  InitialCondition=y0
  Mux : Mux  Inputs=2
  Pad : dspsigops/Pad  padAlong=Columns  dimsToPad=1  valSrc=Specify via dialog  padVal=0  spec=Output size  padNumOutRowsSpecMethod=User-specified  numOutRows=4  padNumOutColsSpecMethod=User-specified  numOutCols=1  isVarDimsMode=off  padBeginning=0  padEnd=0  outSizeMode=User-specified  outSize=1  padSigAt=End  trunc_flag=None  roundingMode=Floor  overflowMode=off  truncOrWrapMode=Truncate  wrap_flag=None
      settings: SourceProductName=DSP System Toolbox  SourceProductBaseCode=DS
  Rate Limiter : RateLimiter  RisingSlewLimit=maxDeltaDot  FallingSlewLimit=-maxDeltaDot  SampleTimeMode=inherited
  Saturation : Saturate  UpperLimit=maxDelta  LowerLimit=-maxDelta
  Scope : Scope  NumInputPorts=4
  Scope1 : Scope
  Sum : Sum  Inputs=|+-
  Sum2 : Sum  Inputs=|+-
  Triggered Subsystem1 : Subsystem  TreatAsAtomicUnit=on
  delta : Outport
  wires:
  Rate Limiter/1 -> Full State Observer/2(delta), Scope1/1, delta/1  "delta"
  Demux2/1 -> Scope/1
  Integrator/1 -> Sum2/2, Pad/1
  Gain1/1 -> Saturation/1
  <r>/1 -> Mux/2
  Full State Observer/1(xhat) -> Sum/2, Demux2/1  "estStates"
  Sum/1 -> Gain1/1
  Pad/1 -> Sum/1
  Mux/1 -> Full State Observer/1(measuredOutputs)
  Demux2/4 -> Scope/4
  Demux2/2 -> Scope/2
  Sum2/1 -> Integrator/1
  Saturation/1 -> Rate Limiter/1
  Demux2/3 -> Scope/3
  Triggered Subsystem1/1(Out1) -> Sum2/1
  <Y>/1 -> Mux/1
  startLaneChange/1 -> Triggered Subsystem1/Trigger
  yRef/1 -> Triggered Subsystem1/1(In1)

== system full_maneuver_platoon_new_strategy/Fd/Regular Vehicle Following ==
  ego : Inport
  leader : Inport  Port=2
  extraSpaceFlag : Inport  Port=3
  Bus Selector : BusSelector  OutputSignals=X,Xdot,u
  Bus Selector1 : BusSelector  OutputSignals=X,Xdot
  Chart : Stateflow chart  BlockKeywords=__PRM__SERIALIZED__DATA__:Stateflow Chart,Stateflow Diagram  TreatAsAtomicUnit=on
  Compare To Constant : simulink/Logic and Bit Operations/Compare To Constant  relop=<  const=5*maxHeadwayError  OutDataTypeStr=boolean
  Compute Errors : Subsystem
  Mux : Mux  Inputs=2
  Rate Limiter : RateLimiter  RisingSlewLimit=maxJerk  FallingSlewLimit=minJerk  SampleTimeMode=inherited
  Rate Limiter1 : RateLimiter  RisingSlewLimit=maxComfJerk  FallingSlewLimit=minComfJerk  SampleTimeMode=inherited
  Scope2 : Scope
  Switch1 : Switch  Criteria=u2 > Threshold
  Veh Following : Subsystem  TreatAsAtomicUnit=on
  Velocity Control : Subsystem  TreatAsAtomicUnit=on
  comf saturation : Saturate  UpperLimit=maxComfAccel  LowerLimit=minComfAccel
  eh : Scope
  output : Scope
  safe saturation : Saturate  UpperLimit=maxAcceleration  LowerLimit=minAcceleration
  veh foll state : Scope  NumInputPorts=2
  u : Outport
  errors : Outport  Port=2
  gap : Outport  Port=3
  leaderInRange : Outport  Port=4
  wires:
  Bus Selector/2 -> Compute Errors/2(vf), Velocity Control/1(velocity)  "<Xdot>"
  Bus Selector/1 -> Compute Errors/1(xf)  "<X>"
  Veh Following/1(u) -> Chart/2(uVehFoll)
  extraSpaceFlag/1 -> Compute Errors/5(extraSpaceFlag)
  Compute Errors/1(eh) -> eh/1, Compare To Constant/1, Veh Following/1(eh), Mux/1
  Compare To Constant/1 -> leaderInRange/1, Chart/1(leaderWithinRange), Veh Following/4(intReset), Velocity Control/3(intReset)
  ego/1 -> Bus Selector/1
  Compute Errors/3("gap ") -> gap/1
  Compute Errors/4(unsafeFlag) -> Switch1/2, Scope2/1
  Rate Limiter1/1 -> Switch1/3  "sat(u)"
  Bus Selector/3 -> Veh Following/3(realInput), Velocity Control/2(realInput)  "<u>"
  Chart/2(u) -> veh foll state/2, safe saturation/1, comf saturation/1
  Switch1/1 -> u/1, output/1
  Rate Limiter/1 -> Switch1/1  "sat(u)"
  safe saturation/1 -> Rate Limiter/1
  comf saturation/1 -> Rate Limiter1/1
  Compute Errors/2(ev) -> Veh Following/2(ev), Mux/2
  Velocity Control/1(u) -> Chart/3(uVelControl)
  Bus Selector1/1 -> Compute Errors/3(xl)  "<X>"
  Mux/1 -> errors/1
  Chart/1(state) -> veh foll state/1
  leader/1 -> Bus Selector1/1
  Bus Selector1/2 -> Compute Errors/4(vl)  "<Xdot>"

== system full_maneuver_platoon_new_strategy/Fd/Subsystem ==
  note: Condition for Lane Changing Vehicle
  note: Condition for Gap Generating Vehicle
  lcFlag : Inport
  ego : Inport  Port=2  OutDataTypeStr=Bus: vehStatesBus
  virtualLeader : Inport  Port=3  OutDataTypeStr=Bus: vehStatesBus
  lcCanStart : Inport  Port=4
  AND : Logic  IconShape=distinctive  AllPortsSameDT=off  OutDataTypeStr=boolean
  AND1 : Logic  IconShape=distinctive  AllPortsSameDT=off  OutDataTypeStr=boolean
  Abs : Abs
  Bus Selector : BusSelector  OutputSignals=Y
  Bus Selector1 : BusSelector  OutputSignals=Y
  Compare To Constant : simulink/Logic and Bit Operations/Compare To Constant  relop=<  const=3.6-0.5  OutDataTypeStr=boolean
  NOT : Logic  Operator=NOT  IconShape=distinctive  AllPortsSameDT=off  OutDataTypeStr=boolean
  OR : Logic  Operator=OR  IconShape=distinctive  AllPortsSameDT=off  OutDataTypeStr=boolean
  Scope : Scope  NumInputPorts=3
  Sum : Sum  Inputs=+-
  lcStarted : Outport
  wires:
  ego/1 -> Bus Selector/1
  virtualLeader/1 -> Bus Selector1/1
  Bus Selector/1 -> Scope/1, Sum/1  "<Y>"
  Bus Selector1/1 -> Scope/2, Sum/2  "<Y>"
  Compare To Constant/1 -> AND1/1
  Sum/1 -> Abs/1
  Abs/1 -> Scope/3, Compare To Constant/1
  lcFlag/1 -> NOT/1, AND/1
  lcCanStart/1 -> AND/2
  NOT/1 -> AND1/2
  OR/1 -> lcStarted/1
  AND1/1 -> OR/1
  AND/1 -> OR/2

== system full_maneuver_platoon_new_strategy/Fd/Subsystem1 ==
  note: Condition for Lane
      | Changing Vehicle
  note: Condition for Gap
      | Generating Vehicle
  ego : Inport  OutDataTypeStr=Bus: vehStatesBus
  futureLeader : Inport  Port=2  OutDataTypeStr=Bus: vehStatesBus
  lcFlag : Inport  Port=3
  AND : Logic  IconShape=distinctive  AllPortsSameDT=off  OutDataTypeStr=boolean
  AND1 : Logic  IconShape=distinctive  AllPortsSameDT=off  OutDataTypeStr=boolean
  Abs : Abs
  Bus Selector1 : BusSelector  OutputSignals=Y
  Bus Selector2 : BusSelector  OutputSignals=Y
  Compare To Constant : simulink/Logic and Bit Operations/Compare To Constant  relop=<=  const=1.8  OutDataTypeStr=boolean
  Compare To Constant1 : simulink/Logic and Bit Operations/Compare To Constant  relop=<=  const=0.5  OutDataTypeStr=boolean
  NOT : Logic  Operator=NOT  IconShape=distinctive  AllPortsSameDT=off  OutDataTypeStr=boolean
  OR : Logic  Operator=OR  IconShape=distinctive  AllPortsSameDT=off  OutDataTypeStr=boolean
  Scope : Scope  NumInputPorts=2
  Sum1 : Sum  Inputs=|+-
  lcDone : Outport
  wires:
  futureLeader/1 -> Bus Selector1/1
  Bus Selector1/1 -> Sum1/2  "<Y>"
  AND/1 -> Scope/1, OR/1
  Compare To Constant/1 -> AND/1
  lcFlag/1 -> AND1/2, NOT/1
  ego/1 -> Bus Selector2/1
  Sum1/1 -> Abs/1
  Compare To Constant1/1 -> AND1/1
  OR/1 -> lcDone/1
  AND1/1 -> Scope/2, OR/2
  Bus Selector2/1 -> Sum1/1  "<Y>"
  Abs/1 -> Compare To Constant1/1, Compare To Constant/1
  NOT/1 -> AND/2

== system full_maneuver_platoon_new_strategy/Fd/Triggered Subsystem ==
  Trigger : TriggerPort  VariantControl=Variant
  Constant : Constant
  Out1 : Outport  InitialOutput=0
  wires:
  Constant/1 -> Out1/1

== system full_maneuver_platoon_new_strategy/Fd/Triggered Subsystem1 ==
  Trigger : TriggerPort  VariantControl=Variant
  Constant : Constant
  Out1 : Outport  InitialOutput=0
  wires:
  Constant/1 -> Out1/1

== system full_maneuver_platoon_new_strategy/Fd/Vehicle Following During LC ==
  ego : Inport
  futureLeader : Inport  Port=2
  extraSpaceFlag : Inport  Port=3
  Enable : EnablePort
  Bus Selector : BusSelector  OutputSignals=X,Xdot,u
  Bus Selector1 : BusSelector  OutputSignals=X,Xdot
  Chart : Stateflow chart  BlockKeywords=__PRM__SERIALIZED__DATA__:Stateflow Chart,Stateflow Diagram  TreatAsAtomicUnit=on
  Compare To Constant : simulink/Logic and Bit Operations/Compare To Constant  relop=<  const=5*maxHeadwayError  OutDataTypeStr=boolean
  Compute Errors : Subsystem
  Mux : Mux  Inputs=2
  Scope : Scope
  Scope3 : Scope
  Terminator : Terminator
  Veh Following : Subsystem  TreatAsAtomicUnit=on
  Velocity Control : Subsystem  TreatAsAtomicUnit=on
  safe acceleration : Saturate  UpperLimit=maxAcceleration  LowerLimit=minAcceleration
  safe jerk : RateLimiter  RisingSlewLimit=maxJerk  FallingSlewLimit=minJerk  SampleTimeMode=inherited
  veh foll state : Scope
  u : Outport  InitialOutput=0
  errors : Outport  Port=2
  gap : Outport  Port=3
  wires:
  futureLeader/1 -> Bus Selector1/1
  Bus Selector/2 -> Velocity Control/1(velocity), Compute Errors/2(vf)  "<Xdot>"
  Compute Errors/1(eh) -> Mux/1, Veh Following/1(eh), Scope/1, Compare To Constant/1
  Compute Errors/4(unsafeFlag) -> Terminator/1
  Chart/1(state) -> veh foll state/1
  Compute Errors/2(ev) -> Veh Following/2(ev), Mux/2
  Bus Selector1/1 -> Compute Errors/3(xl)  "<X>"
  Mux/1 -> errors/1
  extraSpaceFlag/1 -> Compute Errors/5(extraSpaceFlag)
  Bus Selector/3 -> Velocity Control/2(realInput), Veh Following/3(realInput)  "<u>"
  safe jerk/1 -> Scope3/1, u/1  "sat(u)"
  safe acceleration/1 -> safe jerk/1
  Chart/2(u) -> safe acceleration/1
  Velocity Control/1(u) -> Chart/3(uVelControl)
  ego/1 -> Bus Selector/1
  Veh Following/1(u) -> Chart/2(uVehFoll)
  Compare To Constant/1 -> Velocity Control/3(intReset), Veh Following/4(intReset), Chart/1(leaderWithinRange)
  Bus Selector/1 -> Compute Errors/1(xf)  "<X>"
  Compute Errors/3("gap ") -> gap/1
  Bus Selector1/2 -> Compute Errors/4(vl)  "<Xdot>"

== system full_maneuver_platoon_new_strategy/Fd/Virtual Vehicle Following ==
  ego : Inport
  virtualLeader : Inport  Port=2
  extraSpaceFlag : Inport  Port=3
  Enable : EnablePort
  Bus Selector : BusSelector  OutputSignals=X,Xdot,u
  Bus Selector1 : BusSelector  OutputSignals=X,Xdot
  Chart : Stateflow chart  BlockKeywords=__PRM__SERIALIZED__DATA__:Stateflow Chart,Stateflow Diagram  TreatAsAtomicUnit=on
  Compute Errors : Subsystem
  Mux : Mux  Inputs=2
  Scope : Scope
  Sum6 : Sum  Inputs=|+-
  Terminator : Terminator
  Transport Delay1 : TransportDelay  DelayTime=0.01
  Velocity Control : Subsystem  TreatAsAtomicUnit=on
  Virtual Leader Following : Subsystem  TreatAsAtomicUnit=on
  accel saturation : Saturate  UpperLimit=maxComfAccel  LowerLimit=minComfAccel
  jerk saturation : RateLimiter  RisingSlewLimit=maxComfJerk  FallingSlewLimit=minComfJerk  SampleTimeMode=inherited
  vMin : Constant  Value=vMin
  u : Outport  InitialOutput=0
  virtualErrors : Outport  Port=2  OutputWhenDisabled=reset  InitialOutput=[0, 0]
  virtualGap : Outport  Port=3  OutputWhenDisabled=reset  InitialOutput=[0]
  wires:
  Sum6/1 -> Velocity Control/2(ev), Chart/1(velDiff)
  virtualLeader/1 -> Bus Selector1/1
  jerk saturation/1 -> Scope/1, u/1  "virtualFoll"
  Mux/1 -> virtualErrors/1
  vMin/1 -> Sum6/1
  Compute Errors/1(eh) -> Virtual Leader Following/1(eh), Mux/1  "eh"
  Bus Selector/3 -> Virtual Leader Following/3(realInput)  "<u>"
  ego/1 -> Bus Selector/1
  Transport Delay1/1 -> Velocity Control/1(intReset)
  Virtual Leader Following/1(u) -> Chart/3(uVehFoll)  "uVehFoll"
  Bus Selector/2 -> Compute Errors/2(vf), Sum6/2  "<Xdot>"
  accel saturation/1 -> jerk saturation/1
  Bus Selector/1 -> Compute Errors/1(xf)  "<X>"
  Compute Errors/3("gap ") -> virtualGap/1
  Chart/2(u) -> accel saturation/1
  Compute Errors/4(unsafeFlag) -> Terminator/1
  Chart/1(state) -> Transport Delay1/1
  Bus Selector1/1 -> Compute Errors/3(xl)  "<X>"
  Velocity Control/1(Out1) -> Chart/2(uVelControl)  "uVelControl"
  Compute Errors/2(ev) -> Mux/2, Virtual Leader Following/2(ev)
  extraSpaceFlag/1 -> Compute Errors/5(lcFlag)
  Bus Selector1/2 -> Compute Errors/4(vl)  "<Xdot>"

== system full_maneuver_platoon_new_strategy/Fd/followerErrors ==
  ego : Inport
  follower : Inport  Port=2
  Bus Selector1 : BusSelector  OutputSignals=X,Xdot
  Bus Selector3 : BusSelector  OutputSignals=X,Xdot
  Mux : Mux  Inputs=2
  Sum3 : Sum  Inputs=-+|
  Terminator1 : Terminator
  gapToFollower : Subsystem
  errors : Outport
  wires:
  gapToFollower/2("gap ") -> Terminator1/1
  Sum3/1 -> Mux/2
  Bus Selector3/2 -> gapToFollower/2(vf), Sum3/1  "<Xdot>"
  follower/1 -> Bus Selector3/1
  gapToFollower/1(eh) -> Mux/1
  Bus Selector1/2 -> Sum3/2  "<Xdot>"
  Bus Selector3/1 -> gapToFollower/1(xf)  "<X>"
  ego/1 -> Bus Selector1/1
  Bus Selector1/1 -> gapToFollower/3(xl)  "<X>"
  Mux/1 -> errors/1
